simulink model "FixedWingPathDynamics"  (R2021b)
settings: Solver=VariableStepAuto  StartTime=0.0  StopTime=210  RelTol=1e-3
InitFcn:
  | FidelityStage = 2;
model workspace (MAT data in the model file):
  airspeedVal = 12.0293777094
  headingAngles = timeseries
  headingAngles.Name = 'unnamed'
  headingAngles.DataInfo = tsdata.datametadata
  headingAngles.DataInfo.Interpolation = tsdata.interpolation
  headingAngles.DataInfo.Interpolation.Fhandle : function handle (value not decoded)
  headingAngles.DataInfo.Interpolation.Name = 'linear'
  headingAngles.TimeInfo = tsdata.timemetadata
  headingAngles.TimeInfo.Length = 19
  headingAngles.TimeInfo.DuplicateTimes = 0
  headingAngles.TimeInfo.Time_ = [0.1; 0.2; 0.3; 0.4; 0.5; 0.6; 0.7; 0.8; 0.9; 1; 1.1; 1.2; 1.3; 1.4; 1.5; 1.6; 1.7; 1.8; 1.9]
  headingAngles.TimeInfo.Initialized = 1
  headingAngles.QualityInfo = tsdata.qualmetadata
  headingAngles.Data_ = [-0.669202399451; -0.666740658678; -0.663649347949; -0.65999326077; -0.655837190644; -0.651245931077; -0.646284275575; -0.641017017641; -0.635508950781; -0.629824868499; -0.62324164574; -0.615194362721; -0.605985120853; -0.595916021549; -0.585289166221; -0.574406656281; -0.563570593142; -0.553083078215; -0.543246212913]
  lastWaypointInstance = [-187.583573788; -374.036820677; -81.0768]
  lookaheadPoint = timeseries
  lookaheadPoint.Name = 'unnamed'
  lookaheadPoint.DataInfo = tsdata.datametadata
  lookaheadPoint.DataInfo.Interpolation = tsdata.interpolation
  lookaheadPoint.DataInfo.Interpolation.Fhandle : function handle (value not decoded)
  lookaheadPoint.DataInfo.Interpolation.Name = 'linear'
  lookaheadPoint.TimeInfo = tsdata.timemetadata
  lookaheadPoint.TimeInfo.Length = 19
  lookaheadPoint.TimeInfo.DuplicateTimes = 0
  lookaheadPoint.TimeInfo.Time_ = [0.1; 0.2; 0.3; 0.4; 0.5; 0.6; 0.7; 0.8; 0.9; 1; 1.1; 1.2; 1.3; 1.4; 1.5; 1.6; 1.7; 1.8; 1.9]
  lookaheadPoint.TimeInfo.Initialized = 1
  lookaheadPoint.QualityInfo = tsdata.qualmetadata
  lookaheadPoint.Data_ = [-1648.86677503  2025.09037949  482.464791755; -1646.13781659  2022.96170295  482.464791755; -1643.39683878  2020.85041054  482.464791755; -1640.64391692  2018.75673994  482.464791755; -1637.87912629  2016.68092884  482.464791755; -1635.10254219  2014.62321495  482.464791755; -1632.31423992  2012.58383594  482.464791755; -1629.51429479  2010.56302952  482.464791755; -1626.70278208  2008.56103338  482.464791755; -1623.8797771  2006.5780852  482.464791755; -1621.04599578  2004.60930269  482.464791755; -1618.20164622  2002.65137482  482.464791755; -1615.34604196  2000.7068962  482.464791755; -1612.47849657  1998.77846145  482.464791755; -1609.59832358  1996.86866518  482.464791755; -1606.70483656  1994.980102  482.464791755; -1603.79734904  1993.11536653  482.464791755; -1600.8751746  1991.27705337  482.464791755; -1597.93762676  1989.46775715  482.464791755]
  waypointData = [-39.8122089943 -39.8116872817 -39.8111647517 -39.8106414064 -39.8101172475 -39.809592277 -39.8090664968 -39.8085399087 -39.8080125146 -39.8074843164 -39.80695542 -39.8064258792 ... (1797 elements, 599x3)]
undefined symbols (not defined in the file): aircraftTmax, initialThrottle, midFidelityUAV, trimT
libraries: aerolibconvert2 x1, uavalgslib x1
(part 1 of 2)
settings Model: DataDictionary=FideltypathFollowingData.sldd  ModifiedByFormat=The MathWorks, Inc.  SimulationMode=accelerator  PauseTimes=20  Creator=The MathWorks, Inc.  LastModifiedBy=The MathWorks, Inc.
settings DataIOCC: ReturnWorkspaceOutputs=off
settings OptimizationCC: UseDivisionForNetSlopeComputation=UseDivisionForReciprocalsOfIntegersOnly
settings DebuggingCC: AlgebraicLoopMsg=none  ParameterPrecisionLossMsg=none

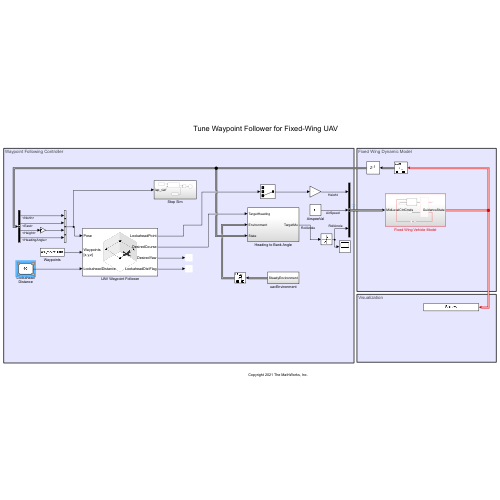
[thumbnail: Simulink's stored preview of the top-level diagram]
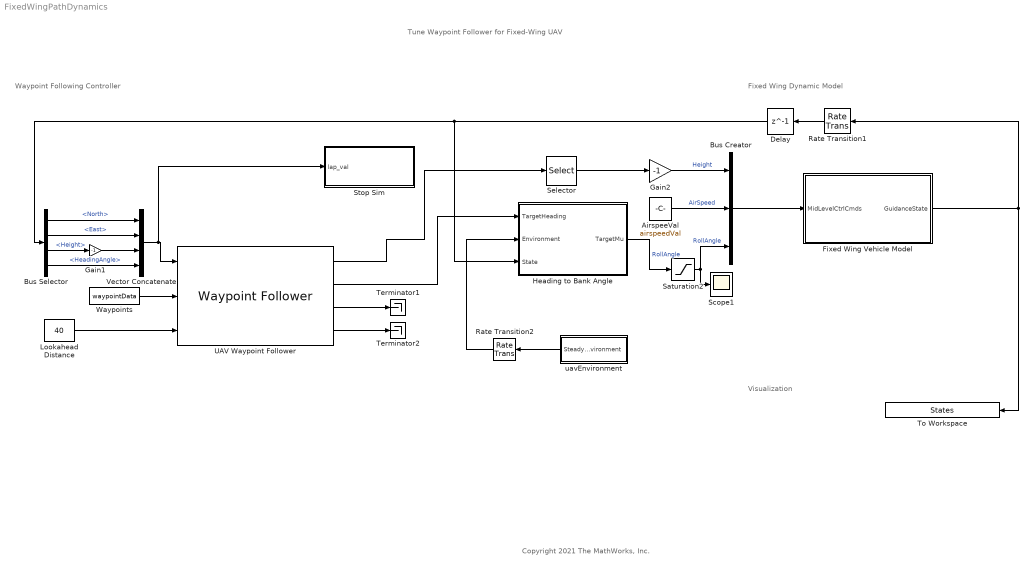
== system FixedWingPathDynamics ==
  note: Copyright 2021 The MathWorks, Inc.
  note: Waypoint Following Controller
  note: Tune Waypoint Follower for Fixed-Wing UAV
  note: Fixed Wing Dynamic Model
  note: Visualization
  AirspeeVal : Constant  Value=airspeedVal  SampleTime=0.01
  Bus Creator : BusCreator  Inputs=3
  Bus Selector : BusSelector  OutputSignals=North,East,Height,HeadingAngle
  Delay : Delay  DelayLength=1  InitialCondition=struct('North', midFidelityUAV.initialNorth, 'East', midFidelityUAV.initialEast,'Height', midFidelityUAV.initialAltitude, 'AirSpeed',midFidelityUAV.initialAirspeed,'HeadingAngle',0,'FlightPathAngle', 0, 'RollAngle',0,'RollAngleRate',0)
  Fixed Wing Vehicle Model : Subsystem  VariantControl=FidelityStage==2
  Gain1 : Gain  Gain=-1
  Gain2 : Gain  Gain=-1
  Heading to Bank Angle : Subsystem
  Lookahead Distance : Constant  Value=40
  Rate Transition1 : RateTransition  OutPortSampleTime=0.01
  Rate Transition2 : RateTransition  OutPortSampleTime=0.01
  Saturation2 : Saturate  UpperLimit=midFidelityUAV.maxroll/180*pi  LowerLimit=-midFidelityUAV.maxroll/180*pi
  Scope1 : Scope
  Selector : Selector  InputPortWidth=3  IndexOptions=Index vector (dialog)  Indices=[3]  OutputSizes=1
  Stop Sim : Subsystem
  Terminator1 : Terminator
  Terminator2 : Terminator
  To Workspace : ToWorkspace  VariableName=States  SaveFormat=Timeseries  SampleTime=0.01
  UAV Waypoint Follower : uavalgslib/Waypoint Follower  UAVType=fixed-wing  StartFrom=first  TransitionRadiusSource=internal  TransitionRadius=10  MinLookaheadDistance=0.1  YawInput=off  ShowCrossTrackErrorOutput=off  ShowStatusOutput=off  SimulateUsing=Code generation
      settings: SourceProductBaseCode=UV
  Vector Concatenate : Concatenate  NumInputs=4
  Waypoints : Constant  Value=waypointData  VectorParams1D=off
  uavEnvironment : Subsystem  VariantControl=NoWind
  wires:
  Rate Transition1/1 -> Delay/1
  AirspeeVal/1 -> Bus Creator/2  "AirSpeed"
  UAV Waypoint Follower/2 -> Heading to Bank Angle/1(TargetHeading)
  UAV Waypoint Follower/1 -> Selector/1
  Bus Selector/4 -> Vector Concatenate/4  "<HeadingAngle>"
  Bus Selector/2 -> Vector Concatenate/2  "<East>"
  Gain1/1 -> Vector Concatenate/3
  Delay/1 -> Heading to Bank Angle/3(State), Bus Selector/1
  Selector/1 -> Gain2/1
  Lookahead Distance/1 -> UAV Waypoint Follower/3
  UAV Waypoint Follower/3 -> Terminator1/1
  UAV Waypoint Follower/4 -> Terminator2/1
  Bus Creator/1 -> Fixed Wing Vehicle Model/1(MidLevelCtrlCmds)
  Bus Selector/1 -> Vector Concatenate/1  "<North>"
  Rate Transition2/1 -> Heading to Bank Angle/2(Environment)
  Fixed Wing Vehicle Model/1(GuidanceState) -> Rate Transition1/1, To Workspace/1
  Bus Selector/3 -> Gain1/1  "<Height>"
  Heading to Bank Angle/1(TargetMu) -> Saturation2/1  "RollAngle"
  Saturation2/1 -> Bus Creator/3, Scope1/1  "RollAngle"
  Gain2/1 -> Bus Creator/1  "Height"
  uavEnvironment/1(SteadyEnvironment) -> Rate Transition2/1
  Waypoints/1 -> UAV Waypoint Follower/2
  Vector Concatenate/1 -> Stop Sim/1(lap_val), UAV Waypoint Follower/1

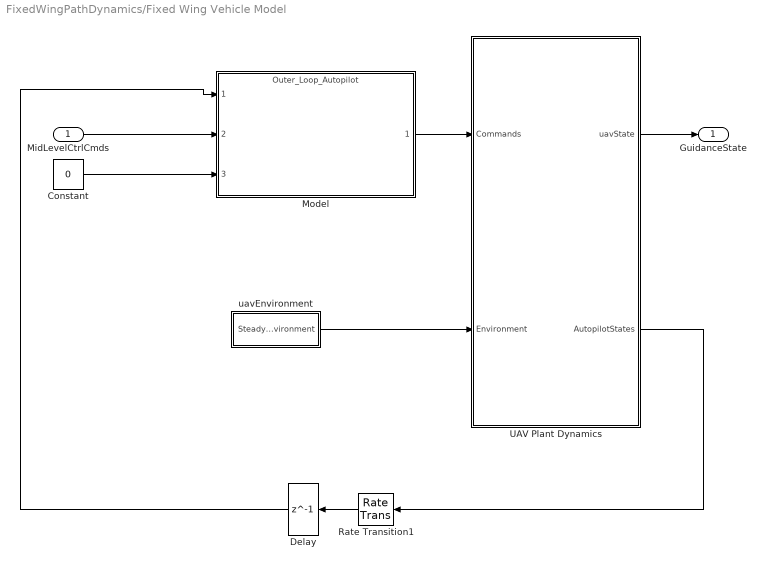
== system FixedWingPathDynamics/Fixed Wing Vehicle Model ==
  MidLevelCtrlCmds : Inport
  Constant : Constant  Value=0
  Delay : Delay  DelayLength=1  InitialCondition=struct('Xe', [0 0 midFidelityUAV.initialAltitude], 'ias',midFidelityUAV.initialAirspeed)  SampleTime=0.01
  Model : ModelReference  ModelNameDialog=Outer_Loop_Autopilot.slx  SimulationMode=Normal  ModelReferenceVersion=2.299
  Rate Transition1 : RateTransition  OutPortSampleTime=0.01
  UAV Plant Dynamics : Subsystem  TreatAsAtomicUnit=on
  uavEnvironment : Subsystem  VariantControl=NoWind
  GuidanceState : Outport
  wires:
  uavEnvironment/1(SteadyEnvironment) -> UAV Plant Dynamics/2(Environment)
  Model/1 -> UAV Plant Dynamics/1(Commands)
  UAV Plant Dynamics/2(AutopilotStates) -> Rate Transition1/1
  UAV Plant Dynamics/1(uavState) -> GuidanceState/1
  Delay/1 -> Model/1
  MidLevelCtrlCmds/1 -> Model/2
  Rate Transition1/1 -> Delay/1
  Constant/1 -> Model/3

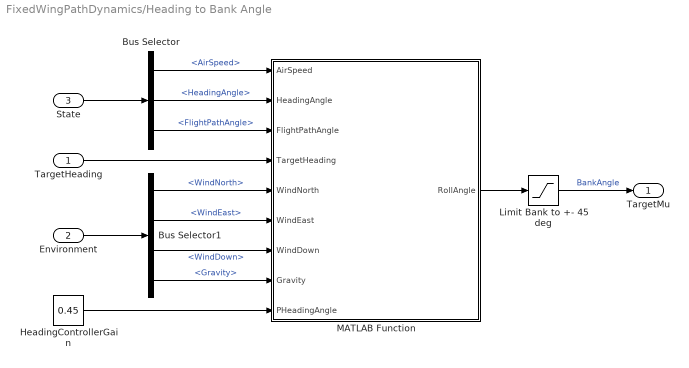
== system FixedWingPathDynamics/Heading to Bank Angle ==
  TargetHeading : Inport  OutDataTypeStr=double  PortDimensions=1
  Environment : Inport  Port=2
  State : Inport  Port=3
  Bus Selector : BusSelector  OutputSignals=AirSpeed,HeadingAngle,FlightPathAngle
  Bus Selector1 : BusSelector  OutputSignals=WindNorth,WindEast,WindDown,Gravity
  HeadingControllerGain : Constant  Value=0.45
  Limit Bank to +- 45 deg : Saturate  UpperLimit=midFidelityUAV.maxroll/180*pi  LowerLimit=-midFidelityUAV.maxroll/180*pi
  MATLAB Function : MATLAB Function  TreatAsAtomicUnit=on
  TargetMu : Outport
  wires:
  Limit Bank to +- 45 deg/1 -> TargetMu/1  "BankAngle"
  Bus Selector1/4 -> MATLAB Function/8(Gravity)  "<Gravity>"
  Bus Selector1/3 -> MATLAB Function/7(WindDown)  "<WindDown>"
  Bus Selector1/2 -> MATLAB Function/6(WindEast)  "<WindEast>"
  Bus Selector1/1 -> MATLAB Function/5(WindNorth)  "<WindNorth>"
  TargetHeading/1 -> MATLAB Function/4(TargetHeading)
  Bus Selector/2 -> MATLAB Function/2(HeadingAngle)  "<HeadingAngle>"
  Bus Selector/1 -> MATLAB Function/1(AirSpeed)  "<AirSpeed>"
  Environment/1 -> Bus Selector1/1
  State/1 -> Bus Selector/1
  HeadingControllerGain/1 -> MATLAB Function/9(PHeadingAngle)
  Bus Selector/3 -> MATLAB Function/3(FlightPathAngle)  "<FlightPathAngle>"
  MATLAB Function/1(RollAngle) -> Limit Bank to +- 45 deg/1

== system FixedWingPathDynamics/Stop Sim ==
  lap_val : Inport
  MATLAB Function : MATLAB Function  TreatAsAtomicUnit=on
  Relational Operator : RelationalOperator  Operator=<=  OutDataTypeStr=boolean  RndMeth=Simplest
  Stop Simulation : Stop
  Waypoints1 : Constant  Value=lastWaypointInstance  VectorParams1D=off
  Waypoints2 : Constant  Value=5  VectorParams1D=off
  wires:
  Waypoints1/1 -> MATLAB Function/1(last_waypoint)
  Relational Operator/1 -> Stop Simulation/1
  MATLAB Function/1(distance) -> Relational Operator/1
  Waypoints2/1 -> Relational Operator/2
  lap_val/1 -> MATLAB Function/2(lap_val)

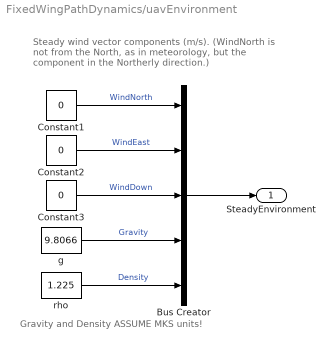
== system FixedWingPathDynamics/uavEnvironment ==
  note: Gravity and Density ASSUME MKS units!
  note: Steady wind vector components (m/s).
      | (WindNorth is not from the North, as in meteorology,
      | but the component in the Northerly direction.)
  Bus Creator : BusCreator  Inputs=5
  Constant1 : Constant  Value=0
  Constant2 : Constant  Value=0
  Constant3 : Constant  Value=0
  g : Constant  Value=9.8066
  rho : Constant  Value=1.225
  SteadyEnvironment : Outport  VectorParamsAs1DForOutWhenUnconnected=off
  wires:
  Constant2/1 -> Bus Creator/2  "WindEast"
  Constant3/1 -> Bus Creator/3  "WindDown"
  Constant1/1 -> Bus Creator/1  "WindNorth"
  Bus Creator/1 -> SteadyEnvironment/1
  g/1 -> Bus Creator/4  "Gravity"
  rho/1 -> Bus Creator/5  "Density"

== system FixedWingPathDynamics/Fixed Wing Vehicle Model/UAV Plant Dynamics ==
  Commands : Inport
  Environment : Inport  Port=2
  Vehicle Dynamics : Subsystem
  asbState to uavState : Subsystem
  uavState : Outport
  AutopilotStates : Outport  Port=2
  wires:
  Vehicle Dynamics/1(AutopilotState) -> asbState to uavState/1(asbState), AutopilotStates/1
  asbState to uavState/1(uavState) -> uavState/1
  Commands/1 -> Vehicle Dynamics/1(Commands)
  Environment/1 -> Vehicle Dynamics/2(Environment)

== system FixedWingPathDynamics/Fixed Wing Vehicle Model/uavEnvironment ==
  note: Gravity and Density ASSUME MKS units!
  note: Steady wind vector components (m/s).
      | (WindNorth is not from the North, as in meteorology,
      | but the component in the Northerly direction.)
  Bus Creator : BusCreator  Inputs=5
  Constant1 : Constant  Value=0
  Constant2 : Constant  Value=0
  Constant3 : Constant  Value=0
  g : Constant  Value=9.8066
  rho : Constant  Value=1.225
  SteadyEnvironment : Outport  VectorParamsAs1DForOutWhenUnconnected=off
  wires:
  Constant2/1 -> Bus Creator/2  "WindEast"
  Constant3/1 -> Bus Creator/3  "WindDown"
  Constant1/1 -> Bus Creator/1  "WindNorth"
  Bus Creator/1 -> SteadyEnvironment/1
  g/1 -> Bus Creator/4  "Gravity"
  rho/1 -> Bus Creator/5  "Density"

== system FixedWingPathDynamics/Fixed Wing Vehicle Model/UAV Plant Dynamics/Vehicle Dynamics ==
  Commands : Inport
  Environment : Inport  Port=2
  AutopilotStates : Subsystem
  Calculate Forces : Subsystem
  Feedback : Subsystem
  Fixed-Wing UAV Point Mass : UAVPointMass  east=midFidelityUAV.initialEast  north=midFidelityUAV.initialNorth  altitude=midFidelityUAV.initialAltitude  airspeed=midFidelityUAV.initialAirspeed  gamma=midFidelityUAV.initialFlightPathAngle  chi=midFidelityUAV.initialHeadingAngle  mass=midFidelityUAV.aircraftM
  AutopilotState : Outport
  wires:
  Calculate Forces/5(gamma_a) -> Fixed-Wing UAV Point Mass/5
  Commands/1 -> Calculate Forces/2(Cmds)
  Calculate Forces/1(Lift) -> Fixed-Wing UAV Point Mass/1
  Feedback/1(Feedback) -> Calculate Forces/1(Feedback)
  AutopilotStates/1(AutopilotStates) -> Feedback/1(AutopilotStates), AutopilotState/1
  Fixed-Wing UAV Point Mass/1 -> AutopilotStates/1(V)
  Fixed-Wing UAV Point Mass/2 -> AutopilotStates/2(G)
  Fixed-Wing UAV Point Mass/3 -> AutopilotStates/3(Va)
  Fixed-Wing UAV Point Mass/4 -> AutopilotStates/4(Ve)
  Fixed-Wing UAV Point Mass/5 -> AutopilotStates/5(XNED)
  Fixed-Wing UAV Point Mass/6 -> AutopilotStates/6(gam_a)
  Fixed-Wing UAV Point Mass/7 -> AutopilotStates/7(gam)
  Fixed-Wing UAV Point Mass/8 -> AutopilotStates/8(chi_a)
  Environment/1 -> Calculate Forces/3(Environment)
  Calculate Forces/2(Drag) -> Fixed-Wing UAV Point Mass/2
  Calculate Forces/3(Weight1) -> Fixed-Wing UAV Point Mass/3
  Calculate Forces/4(Thrust1) -> Fixed-Wing UAV Point Mass/4
  Calculate Forces/6(mu) -> Fixed-Wing UAV Point Mass/6, AutopilotStates/10(mu)
  Calculate Forces/8(WindVector) -> Fixed-Wing UAV Point Mass/8
  Calculate Forces/7(alpha) -> Fixed-Wing UAV Point Mass/7
  Fixed-Wing UAV Point Mass/9 -> AutopilotStates/9(chi)

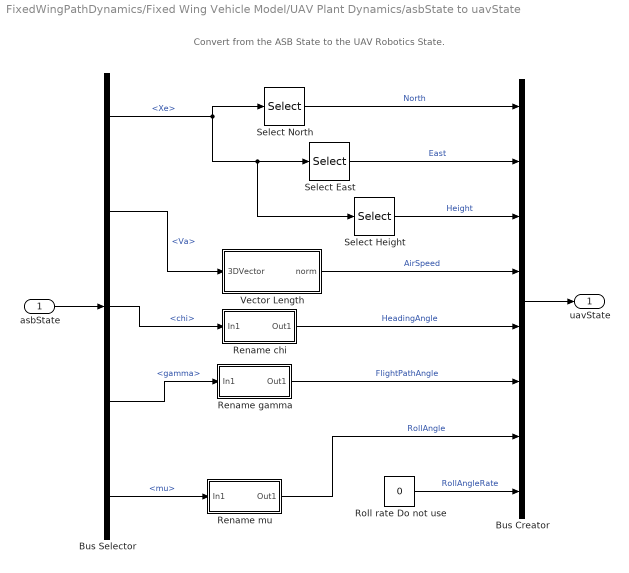
== system FixedWingPathDynamics/Fixed Wing Vehicle Model/UAV Plant Dynamics/asbState to uavState ==
  note: Convert from the ASB State to the UAV Robotics State.
  asbState : Inport
  Bus Creator : BusCreator  Inputs=8
  Bus Selector : BusSelector  OutputSignals=Xe,Va,chi,gamma,mu
  Rename chi : Subsystem
  Rename gamma : Subsystem
  Rename mu : Subsystem
  Roll rate Do not use : Constant  Value=0
  Select East : Selector  InputPortWidth=3  IndexOptions=Index vector (dialog)  Indices=[2]  OutputSizes=1
  Select Height : Selector  InputPortWidth=3  IndexOptions=Index vector (dialog)  Indices=[3]  OutputSizes=1
  Select North : Selector  InputPortWidth=3  IndexOptions=Index vector (dialog)  Indices=[1]  OutputSizes=1
  Vector Length : Subsystem
  uavState : Outport
  wires:
  Bus Selector/3 -> Rename chi/1(In1)  "<chi>"
  Bus Selector/4 -> Rename gamma/1(In1)  "<gamma>"
  Bus Selector/5 -> Rename mu/1(In1)  "<mu>"
  asbState/1 -> Bus Selector/1
  Bus Creator/1 -> uavState/1
  Bus Selector/1 -> Select Height/1, Select East/1, Select North/1  "<Xe>"
  Select East/1 -> Bus Creator/2  "East"
  Select North/1 -> Bus Creator/1  "North"
  Select Height/1 -> Bus Creator/3  "Height"
  Bus Selector/2 -> Vector Length/1(3DVector)  "<Va>"
  Vector Length/1(norm) -> Bus Creator/4  "AirSpeed"
  Rename gamma/1(Out1) -> Bus Creator/6  "FlightPathAngle"
  Rename chi/1(Out1) -> Bus Creator/5  "HeadingAngle"
  Rename mu/1(Out1) -> Bus Creator/7  "RollAngle"
  Roll rate Do not use/1 -> Bus Creator/8  "RollAngleRate"

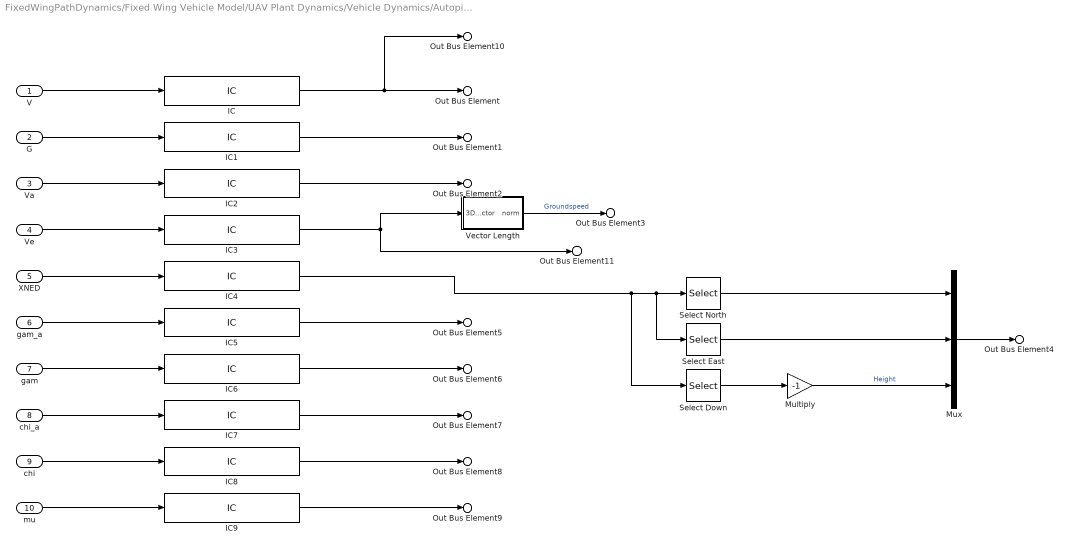
== system FixedWingPathDynamics/Fixed Wing Vehicle Model/UAV Plant Dynamics/Vehicle Dynamics/AutopilotStates ==
  V : Inport
  G : Inport  Port=2
  Va : Inport  Port=3
  Ve : Inport  Port=4
  XNED : Inport  Port=5
  gam_a : Inport  Port=6
  gam : Inport  Port=7
  chi_a : Inport  Port=8
  chi : Inport  Port=9
  mu : Inport  Port=10
  IC : InitialCondition  Value=midFidelityUAV.initialAirspeed
  IC1 : InitialCondition  Value=midFidelityUAV.initialAirspeed
  IC2 : InitialCondition  Value=[midFidelityUAV.initialAirspeed 0 0]
  IC3 : InitialCondition  Value=[midFidelityUAV.initialAirspeed 0 0 ]
  IC4 : InitialCondition  Value=[midFidelityUAV.initialNorth midFidelityUAV.initialEast midFidelityUAV.initialAltitude]
  IC5 : InitialCondition  Value=midFidelityUAV.initialFlightPathAngle
  IC6 : InitialCondition  Value=midFidelityUAV.initialFlightPathAngle
  IC7 : InitialCondition  Value=midFidelityUAV.initialHeadingAngle
  IC8 : InitialCondition  Value=midFidelityUAV.initialHeadingAngle
  IC9 : InitialCondition  Value=0
  Multiply : Gain  Gain=-1
  Mux : Mux  Inputs=3
  Select Down : Selector  InputPortWidth=3  IndexOptions=Index vector (dialog)  Indices=[3]  OutputSizes=1
  Select East : Selector  InputPortWidth=3  IndexOptions=Index vector (dialog)  Indices=[2]  OutputSizes=1
  Select North : Selector  InputPortWidth=3  IndexOptions=Index vector (dialog)  Indices=[1]  OutputSizes=1
  Vector Length : Subsystem
  Out Bus Element : Outport  PortName=AutopilotStates  Element=V
  Out Bus Element1 : Outport  PortName=AutopilotStates  Element=G
  Out Bus Element2 : Outport  PortName=AutopilotStates  Element=Va
  Out Bus Element3 : Outport  PortName=AutopilotStates  Element=GS
  Out Bus Element4 : Outport  PortName=AutopilotStates  Element=Xe
  Out Bus Element5 : Outport  PortName=AutopilotStates  Element=gamma_a
  Out Bus Element6 : Outport  PortName=AutopilotStates  Element=gamma
  Out Bus Element7 : Outport  PortName=AutopilotStates  Element=chi_a
  Out Bus Element8 : Outport  PortName=AutopilotStates  Element=chi
  Out Bus Element9 : Outport  PortName=AutopilotStates  Element=mu
  Out Bus Element10 : Outport  PortName=AutopilotStates  Element=ias
  Out Bus Element11 : Outport  PortName=AutopilotStates  Element=Ve
  wires:
  IC8/1 -> Out Bus Element8/1
  mu/1 -> IC9/1
  Vector Length/1(norm) -> Out Bus Element3/1  "Groundspeed"
  V/1 -> IC/1
  IC/1 -> Out Bus Element/1, Out Bus Element10/1
  G/1 -> IC1/1
  Va/1 -> IC2/1
  Ve/1 -> IC3/1
  XNED/1 -> IC4/1
  gam_a/1 -> IC5/1
  gam/1 -> IC6/1
  chi_a/1 -> IC7/1
  chi/1 -> IC8/1
  IC1/1 -> Out Bus Element1/1
  IC2/1 -> Out Bus Element2/1
  IC3/1 -> Vector Length/1(3DVector), Out Bus Element11/1
  IC4/1 -> Select Down/1, Select East/1, Select North/1
  IC5/1 -> Out Bus Element5/1
  IC6/1 -> Out Bus Element6/1
  IC7/1 -> Out Bus Element7/1
  Select Down/1 -> Multiply/1
  Select North/1 -> Mux/1
  Select East/1 -> Mux/2
  Multiply/1 -> Mux/3  "Height"
  Mux/1 -> Out Bus Element4/1
  IC9/1 -> Out Bus Element9/1

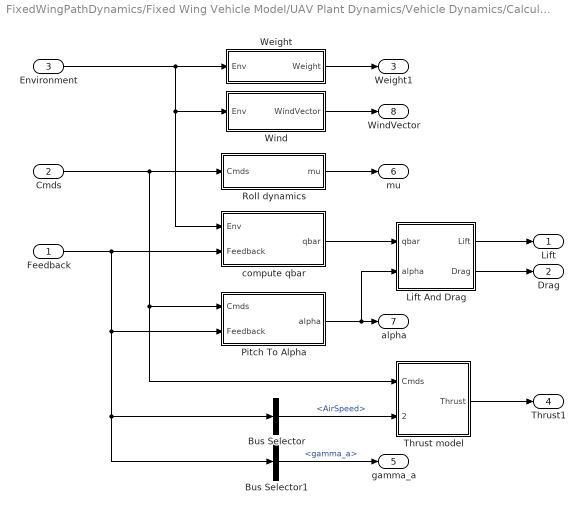
== system FixedWingPathDynamics/Fixed Wing Vehicle Model/UAV Plant Dynamics/Vehicle Dynamics/Calculate Forces ==
  Feedback : Inport
  Cmds : Inport  Port=2
  Environment : Inport  Port=3
  Bus Selector : BusSelector  OutputSignals=AirSpeed
  Bus Selector1 : BusSelector  OutputSignals=gamma_a
  Lift And Drag : Subsystem
  Pitch To Alpha : Subsystem
  Roll dynamics : Subsystem
  Thrust model : Subsystem  Variant=on  VariantControlMode=label  VariantControl=Choice  LabelModeActiveChoice=ThrustAd==1
  Weight : Subsystem
  Wind : Subsystem
  compute qbar : Subsystem
  Lift : Outport
  Drag : Outport  Port=2
  Weight1 : Outport  Port=3
  Thrust1 : Outport  Port=4
  gamma_a : Outport  Port=5
  mu : Outport  Port=6
  alpha : Outport  Port=7
  WindVector : Outport  Port=8
  wires:
  Thrust model/1(Thrust) -> Thrust1/1
  Lift And Drag/1(Lift) -> Lift/1
  Lift And Drag/2(Drag) -> Drag/1
  Wind/1(WindVector) -> WindVector/1
  Bus Selector/1 -> Thrust model/2(Airspeed)  "<AirSpeed>"
  compute qbar/1(qbar) -> Lift And Drag/1(qbar)
  Weight/1(Weight) -> Weight1/1
  Roll dynamics/1(mu) -> mu/1
  Bus Selector1/1 -> gamma_a/1  "<gamma_a>"
  Environment/1 -> compute qbar/1(Env), Wind/1(Env), Weight/1(Env)
  Cmds/1 -> Thrust model/1(Cmds), Pitch To Alpha/1(Cmds), Roll dynamics/1(Cmds)
  Feedback/1 -> Bus Selector/1, Bus Selector1/1, Pitch To Alpha/2(Feedback), compute qbar/2(Feedback)
  Pitch To Alpha/1(alpha) -> alpha/1, Lift And Drag/2(alpha)

== system FixedWingPathDynamics/Fixed Wing Vehicle Model/UAV Plant Dynamics/Vehicle Dynamics/Feedback ==
  In Bus Element : Inport  PortName=AutopilotStates  Element=G
  In Bus Element1 : Inport  PortName=AutopilotStates  Element=V
  In Bus Element2 : Inport  PortName=AutopilotStates  Element=gamma_a
  Out Bus Element : Outport  PortName=Feedback  Element=GroundSpeed
  Out Bus Element1 : Outport  PortName=Feedback  Element=AirSpeed
  Out Bus Element2 : Outport  PortName=Feedback  Element=gamma_a
  wires:
  In Bus Element2/1 -> Out Bus Element2/1
  In Bus Element1/1 -> Out Bus Element1/1
  In Bus Element/1 -> Out Bus Element/1

== system FixedWingPathDynamics/Fixed Wing Vehicle Model/UAV Plant Dynamics/asbState to uavState/Rename chi ==
  In1 : Inport
  Out1 : Outport
  wires:
  In1/1 -> Out1/1

== system FixedWingPathDynamics/Fixed Wing Vehicle Model/UAV Plant Dynamics/asbState to uavState/Rename gamma ==
  In1 : Inport
  Out1 : Outport
  wires:
  In1/1 -> Out1/1

== system FixedWingPathDynamics/Fixed Wing Vehicle Model/UAV Plant Dynamics/asbState to uavState/Rename mu ==
  In1 : Inport
  Out1 : Outport
  wires:
  In1/1 -> Out1/1

== system FixedWingPathDynamics/Fixed Wing Vehicle Model/UAV Plant Dynamics/asbState to uavState/Vector Length ==
  3DVector : Inport
  Add : Sum  Inputs=+
  Square : Math  Operator=square  SaturateOnIntegerOverflow=on
  Square Root : Sqrt  SaturateOnIntegerOverflow=on
  norm : Outport
  wires:
  Square Root/1 -> norm/1
  Add/1 -> Square Root/1
  Square/1 -> Add/1
  3DVector/1 -> Square/1

== system FixedWingPathDynamics/Fixed Wing Vehicle Model/UAV Plant Dynamics/Vehicle Dynamics/AutopilotStates/Vector Length ==
  3DVector : Inport
  Add : Sum  Inputs=+
  Square : Math  Operator=square  SaturateOnIntegerOverflow=on
  Square Root : Sqrt  SaturateOnIntegerOverflow=on
  norm : Outport
  wires:
  Square Root/1 -> norm/1
  Add/1 -> Square Root/1
  Square/1 -> Add/1
  3DVector/1 -> Square/1

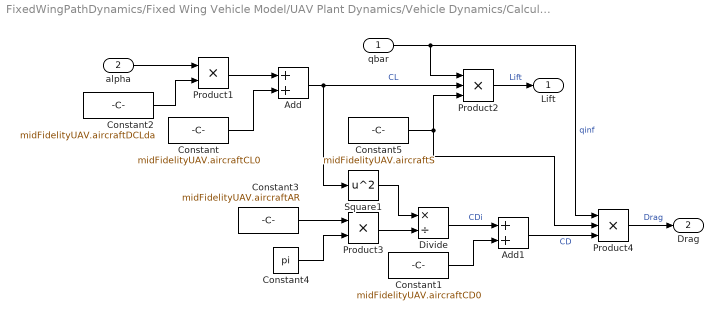
== system FixedWingPathDynamics/Fixed Wing Vehicle Model/UAV Plant Dynamics/Vehicle Dynamics/Calculate Forces/Lift And Drag ==
  qbar : Inport
  alpha : Inport  Port=2
  Add : Sum
  Add1 : Sum
  Constant : Constant  Value=midFidelityUAV.aircraftCL0
  Constant1 : Constant  Value=midFidelityUAV.aircraftCD0
  Constant2 : Constant  Value=midFidelityUAV.aircraftDCLda
  Constant3 : Constant  Value=midFidelityUAV.aircraftAR
  Constant4 : Constant  Value=pi
  Constant5 : Constant  Value=midFidelityUAV.aircraftS
  Divide : Product  Inputs=*/
  Product1 : Product
  Product2 : Product  Inputs=3
  Product3 : Product
  Product4 : Product  Inputs=3
  Square1 : Math  Operator=square  SaturateOnIntegerOverflow=on
  Lift : Outport
  Drag : Outport  Port=2
  wires:
  qbar/1 -> Product4/1, Product2/1  "qinf"
  alpha/1 -> Product1/1
  Constant2/1 -> Product1/2
  Product1/1 -> Add/1
  Constant/1 -> Add/2
  Add/1 -> Product2/2, Square1/1  "CL"
  Constant5/1 -> Product2/3, Product4/2
  Product2/1 -> Lift/1  "Lift"
  Constant3/1 -> Product3/1
  Constant4/1 -> Product3/2
  Product3/1 -> Divide/2
  Square1/1 -> Divide/1
  Divide/1 -> Add1/1  "CDi"
  Constant1/1 -> Add1/2
  Add1/1 -> Product4/3  "CD"
  Product4/1 -> Drag/1  "Drag"

== system FixedWingPathDynamics/Fixed Wing Vehicle Model/UAV Plant Dynamics/Vehicle Dynamics/Calculate Forces/Pitch To Alpha ==
  note: Pitch=alpha+gamma_a
  Cmds : Inport
  Feedback : Inport  Port=2
  Add : Sum  Inputs=+-
  Bus Selector : BusSelector  OutputSignals=Pitch
  Bus Selector1 : BusSelector  OutputSignals=gamma_a
  alpha : Outport
  wires:
  Add/1 -> alpha/1
  Bus Selector1/1 -> Add/2  "<gamma_a>"
  Feedback/1 -> Bus Selector1/1
  Bus Selector/1 -> Add/1  "<Pitch>"
  Cmds/1 -> Bus Selector/1

== system FixedWingPathDynamics/Fixed Wing Vehicle Model/UAV Plant Dynamics/Vehicle Dynamics/Calculate Forces/Roll dynamics ==
  Cmds : Inport
  Bus Selector1 : BusSelector  OutputSignals=Roll
  Saturation2 : Saturate  UpperLimit=midFidelityUAV.maxroll/180*pi  LowerLimit=-midFidelityUAV.maxroll/180*pi
  Transfer Fcn1 : TransferFcn  Numerator=5.448  Denominator=[1 4.6668 5.448]
  mu : Outport
  wires:
  Bus Selector1/1 -> Transfer Fcn1/1  "<Roll>"
  Cmds/1 -> Bus Selector1/1
  Saturation2/1 -> mu/1
  Transfer Fcn1/1 -> Saturation2/1

== system FixedWingPathDynamics/Fixed Wing Vehicle Model/UAV Plant Dynamics/Vehicle Dynamics/Calculate Forces/Thrust model ==
  Cmds : Inport
  Airspeed : Inport  Port=2
  Advanced : Subsystem  VariantControl=ThrustAd==1
  "Simple " : Subsystem  VariantControl=ThrustAd==0
  Thrust : Outport

== system FixedWingPathDynamics/Fixed Wing Vehicle Model/UAV Plant Dynamics/Vehicle Dynamics/Calculate Forces/Weight ==
  Env : Inport
  Bus Selector : BusSelector  OutputSignals=Gravity
  Constant1 : Constant  Value=midFidelityUAV.aircraftM
  Product : Product
  Weight : Outport
  wires:
  Bus Selector/1 -> Product/1  "<Gravity>"
  Constant1/1 -> Product/2
  Product/1 -> Weight/1
  Env/1 -> Bus Selector/1

== system FixedWingPathDynamics/Fixed Wing Vehicle Model/UAV Plant Dynamics/Vehicle Dynamics/Calculate Forces/Wind ==
  Env : Inport
  Bus Creator1 : BusCreator  Inputs=3
  Bus Selector1 : BusSelector  OutputSignals=WindNorth,WindEast,WindDown
  Bus to Vector : BusToVector
  WindVector : Outport
  wires:
  Env/1 -> Bus Selector1/1
  Bus Selector1/3 -> Bus Creator1/3  "<WindDown>"
  Bus Selector1/2 -> Bus Creator1/2  "<WindEast>"
  Bus Selector1/1 -> Bus Creator1/1  "<WindNorth>"
  Bus Creator1/1 -> Bus to Vector/1
  Bus to Vector/1 -> WindVector/1

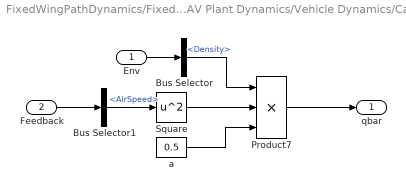
== system FixedWingPathDynamics/Fixed Wing Vehicle Model/UAV Plant Dynamics/Vehicle Dynamics/Calculate Forces/compute qbar ==
  Env : Inport
  Feedback : Inport  Port=2
  Bus Selector : BusSelector  OutputSignals=Density
  Bus Selector1 : BusSelector  OutputSignals=AirSpeed
  Product7 : Product  Inputs=3
  Square : Math  Operator=square  SaturateOnIntegerOverflow=on
  a : Constant  Value=0.5
  qbar : Outport  OutDataTypeStr=double  PortDimensions=1
  wires:
  Bus Selector1/1 -> Square/1  "<AirSpeed>"
  Feedback/1 -> Bus Selector1/1
  Product7/1 -> qbar/1
  Bus Selector/1 -> Product7/1  "<Density>"
  Env/1 -> Bus Selector/1
  a/1 -> Product7/3
  Square/1 -> Product7/2

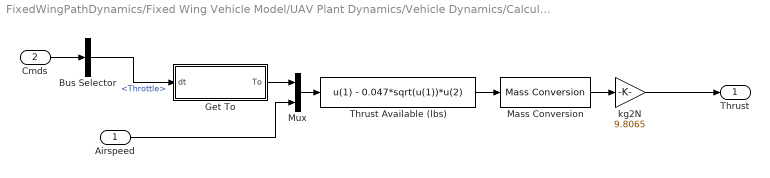
== system FixedWingPathDynamics/Fixed Wing Vehicle Model/UAV Plant Dynamics/Vehicle Dynamics/Calculate Forces/Thrust model/Advanced ==
  Airspeed : Inport
  Cmds : Inport  Port=2
  Bus Selector : BusSelector  OutputSignals=Throttle
  Get To : Subsystem
  Mass Conversion : aerolibconvert2/Mass Conversion  IU=lbm  OU=kg
      settings: SourceProductBaseCode=AE
  Mux : Mux  Inputs=2
  Thrust Available (lbs) : Fcn  Expr=u(1) - 0.047*sqrt(u(1))*u(2)
  kg2N : Gain  Gain=9.8065  SaturateOnIntegerOverflow=on  OutDataTypeStr=Inherit: Same as input  ParamDataTypeStr=Inherit: Same as input
      settings: AttributesFormatString=%<Gain>
  Thrust : Outport  Unit=kg*m/s^2  VectorParamsAs1DForOutWhenUnconnected=off
  wires:
  Cmds/1 -> Bus Selector/1
  Bus Selector/1 -> Get To/1(dt)  "<Throttle>"
  Get To/1(To) -> Mux/1
  Mux/1 -> Thrust Available (lbs)/1
  Thrust Available (lbs)/1 -> Mass Conversion/1
  Airspeed/1 -> Mux/2
  kg2N/1 -> Thrust/1
  Mass Conversion/1 -> kg2N/1

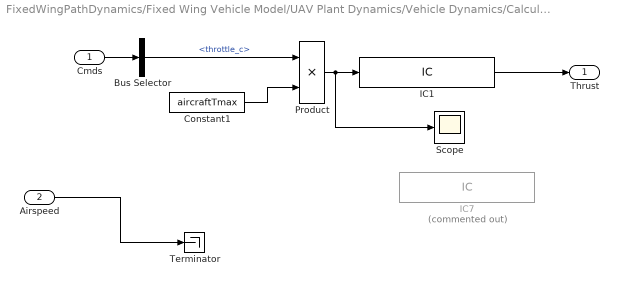
== system FixedWingPathDynamics/Fixed Wing Vehicle Model/UAV Plant Dynamics/Vehicle Dynamics/Calculate Forces/Thrust model/Simple  ==
  Cmds : Inport
  Airspeed : Inport  Port=2
  Bus Selector : BusSelector  OutputSignals=throttle_c
  Constant1 : Constant  Value=aircraftTmax
  IC1 : InitialCondition  Value=trimT
  IC7 : InitialCondition  Commented=on  Value=initialThrottle*aircraftTmax
  Product : Product
  Scope : Scope
  Terminator : Terminator
  Thrust : Outport
  wires:
  Airspeed/1 -> Terminator/1
  Bus Selector/1 -> Product/1  "<throttle_c>"
  IC1/1 -> Thrust/1
  Cmds/1 -> Bus Selector/1
  Constant1/1 -> Product/2
  Product/1 -> IC1/1, Scope/1
